simulink model "lab1s2022a"  (R2022b)
settings: Solver=VariableStepAuto  StartTime=0.0  StopTime=Tmdl*0.2  MaxStep=0.001  RelTol=1e-3
undefined symbols (not defined in the file): b12, dfi, J1, J2, k12, Ke, KT, Ra, T1, T2, Ta, Tref, Ua
libraries: slctrlblks x3
settings Model: Creator=81502  LastModifiedBy=86156
settings ModelReferenceCC: EnableRefExpFcnMdlSchedulingChecks=on

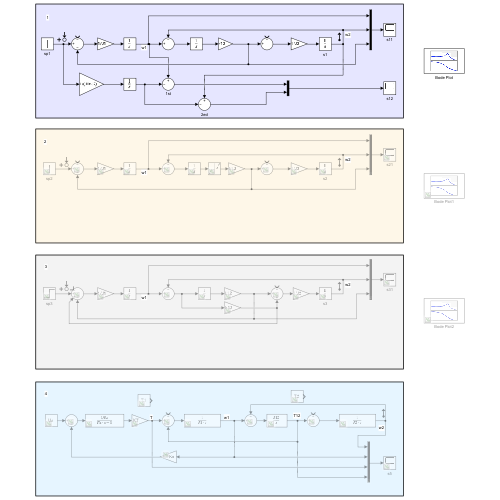
[thumbnail: Simulink's stored preview of the top-level diagram]
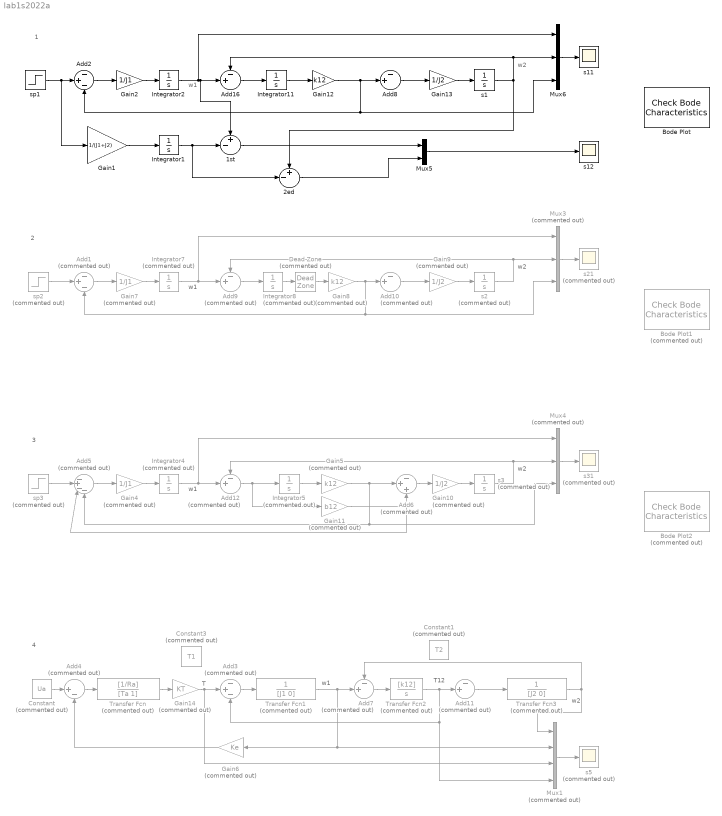
== system lab1s2022a ==
  note: T12
  note: w1
  note: T
  note: 3
  note: 2
  note: 1
  note: w2
  note: w1
  note: w1
  note: w2
  note: w1
  note: w2
  note: 4
  note: w2
  1st : Sum  Inputs=+-|
  2ed : Sum  Inputs=+-|
  Add1 : Sum  Commented=on  Inputs=-+-
  Add{7,9..12} (5 alike) : Sum  Commented=on  Inputs=-+|
  Add16 : Sum  Inputs=-+|
  Add2 : Sum  Inputs=-+-
  Add3 : Sum  Commented=on  Inputs=-+-
  Add4 : Sum  Commented=on  Inputs=|+-
  Add5 : Sum  Commented=on  Inputs=|-+--
  Add6 : Sum  Commented=on  Inputs=-++
  Add8 : Sum  Inputs=-+|
  Bode Plot : slctrlblks/Model Verification/Check Bode  Characteristics  InstantiateOnLoad=on  SaveOperatingPoints=off  LinearizationIOs={'/sp1', 1, 'in', 'off', '';'/s1', 1, 'out', 'off', ''}  LinearizeAt=SnapshotTimes  SnapshotTimes=[0]  TriggerType=rising  SampleTime=auto  RateConversionMethod=zoh  PreWarpFreq=10  UseExactDelayModel=off  UseFullBlockNameLabels=off  UseBusSignalLabels=off  enabled=on  stopWhenAssertionFail=off  export=off  ViewDlgPos=[1264.33333333333 431.666666666667 864 493.333333333333]  OpenViewOnLoad=off  LaunchViewOnOpen=on  FrequencyUnits=rad/s  MagnitudeUnits=dB  PhaseUnits=deg  TimeUnits=seconds  EnableUpperBound=off  UpperBoundFrequencies=[]  UpperBoundMagnitudes=[]  EnableLowerBound=off  LowerBoundFrequencies=[]  LowerBoundMagnitudes=[]
  Bode Plot1 : slctrlblks/Model Verification/Check Bode  Characteristics  Commented=on  InstantiateOnLoad=on  SaveOperatingPoints=off  LinearizationIOs={'/sp2', 1, 'in', 'off', '';'/s2', 1, 'out', 'off', ''}  LinearizeAt=SnapshotTimes  SnapshotTimes=[0]  TriggerType=rising  SampleTime=auto  RateConversionMethod=zoh  PreWarpFreq=10  UseExactDelayModel=off  UseFullBlockNameLabels=off  UseBusSignalLabels=off  enabled=on  stopWhenAssertionFail=off  export=off  ViewDlgPos=[1489 63.6666666666667 620 384]  OpenViewOnLoad=off  LaunchViewOnOpen=on  FrequencyUnits=rad/s  MagnitudeUnits=dB  PhaseUnits=deg  TimeUnits=seconds  EnableUpperBound=off  UpperBoundFrequencies=[]  UpperBoundMagnitudes=[]  EnableLowerBound=off  LowerBoundFrequencies=[]  LowerBoundMagnitudes=[]
  Bode Plot2 : slctrlblks/Model Verification/Check Bode  Characteristics  Commented=on  InstantiateOnLoad=on  SaveOperatingPoints=off  LinearizationIOs={'/sp3', 1, 'in', 'off', '';'/s3', 1, 'out', 'off', ''}  LinearizeAt=SnapshotTimes  SnapshotTimes=[0]  TriggerType=rising  SampleTime=auto  RateConversionMethod=zoh  PreWarpFreq=10  UseExactDelayModel=off  UseFullBlockNameLabels=off  UseBusSignalLabels=off  enabled=on  stopWhenAssertionFail=off  export=off  ViewDlgPos=[1489 63.6666666666667 620 384]  OpenViewOnLoad=off  LaunchViewOnOpen=on  FrequencyUnits=rad/s  MagnitudeUnits=dB  PhaseUnits=deg  TimeUnits=seconds  EnableUpperBound=off  UpperBoundFrequencies=[]  UpperBoundMagnitudes=[]  EnableLowerBound=off  LowerBoundFrequencies=[]  LowerBoundMagnitudes=[]
  Constant : Constant  Commented=on  Value=Ua
  Constant1 : Constant  Commented=on  Value=T2
  Constant3 : Constant  Commented=on  Value=T1
  Dead Zone : DeadZone  Commented=on  LowerValue=-dfi/2  UpperValue=dfi/2
  Gain1 : Gain  Gain=1/(J1+J2)
  Gain10 : Gain  Commented=on  Gain=1/J2
  Gain11 : Gain  Commented=on  Gain=b12
  Gain12 : Gain  Gain=k12
  Gain13 : Gain  Gain=1/J2
  Gain14 : Gain  Commented=on  Gain=KT
  Gain2 : Gain  Gain=1/J1
  Gain4 : Gain  Commented=on  Gain=1/J1
  Gain5 : Gain  Commented=on  Gain=k12
  Gain6 : Gain  Commented=on  Gain=Ke
  Gain7 : Gain  Commented=on  Gain=1/J1
  Gain8 : Gain  Commented=on  Gain=k12
  Gain9 : Gain  Commented=on  Gain=1/J2
  Integrator1 : Integrator
  Integrator11 : Integrator
  Integrator2 : Integrator
  Integrator{4..5,7..8} (4 alike) : Integrator  Commented=on
  Mux1 : Mux  Commented=on
  Mux3 : Mux  Commented=on  Inputs=3
  Mux4 : Mux  Commented=on  Inputs=3
  Mux5 : Mux  Inputs=2
  Mux6 : Mux  Inputs=3
  Transfer Fcn : TransferFcn  Commented=on  Numerator=[1/Ra]  Denominator=[Ta 1]
  Transfer Fcn1 : TransferFcn  Commented=on  Denominator=[J1 0]
  Transfer Fcn2 : TransferFcn  Commented=on  Numerator=[k12]  Denominator=[1 0]
  Transfer Fcn3 : TransferFcn  Commented=on  Denominator=[J2 0]
  s1 : Integrator
  s11 : Scope
  s12 : Scope
  s2 : Integrator  Commented=on
  s21 : Scope  Commented=on
  s3 : Integrator  Commented=on
  s31 : Scope  Commented=on
  s5 : Scope  Commented=on
  sp1 : Step  Time=0.1  After=Tref  SampleTime=0
  sp2 : Step  Commented=on  Time=0.1  After=0.1*Tref  SampleTime=0
  sp3 : Step  Commented=on  Time=0.1  After=Tref  SampleTime=0
  wires:
  s2/1 -> Add9/1, Mux3/2
  Add9/1 -> Integrator8/1
  Gain7/1 -> Integrator7/1
  Add10/1 -> Gain9/1
  Gain8/1 -> Add10/2, Add1/3, Mux3/3
  Gain9/1 -> s2/1
  Add1/1 -> Gain7/1
  Mux3/1 -> s21/1
  Integrator7/1 -> Add9/2, Mux3/1
  sp2/1 -> Add1/2
  Gain5/1 -> Add5/4, Mux4/3, Add6/2
  Mux4/1 -> s31/1
  Gain10/1 -> s3/1
  Gain4/1 -> Integrator4/1
  Add12/1 -> Gain11/1, Integrator5/1
  sp3/1 -> Add5/2
  Integrator5/1 -> Gain5/1
  s3/1 -> Add12/1, Mux4/2
  Add6/1 -> Gain10/1
  Add5/1 -> Gain4/1
  Integrator4/1 -> Add12/2, Mux4/1
  Gain11/1 -> Add6/3, Add5/3
  Add16/1 -> Integrator11/1
  Integrator11/1 -> Gain12/1
  Mux6/1 -> s11/1
  Gain13/1 -> s1/1
  Gain2/1 -> Integrator2/1
  sp1/1 -> Add2/2, Gain1/1
  s1/1 -> 2ed/1, Add16/1, Mux6/2
  Gain12/1 -> Add8/2, Add2/3, Mux6/3
  Add8/1 -> Gain13/1
  1st/1 -> Mux5/1
  2ed/1 -> Mux5/2
  Add2/1 -> Gain2/1
  Gain1/1 -> Integrator1/1
  Integrator1/1 -> 2ed/2, 1st/2
  Integrator2/1 -> Add16/2, 1st/1, Mux6/1
  Mux5/1 -> s12/1
  Dead Zone/1 -> Gain8/1
  Integrator8/1 -> Dead Zone/1
  Add3/1 -> Transfer Fcn1/1
  Add7/1 -> Transfer Fcn2/1
  Gain14/1 -> Add3/2, Mux1/3
  Transfer Fcn2/1 -> Add11/2, Add3/3, Mux1/4
  Constant/1 -> Add4/1
  Mux1/1 -> s5/1
  Transfer Fcn1/1 -> Add7/2, Gain6/1, Mux1/2
  Add4/1 -> Transfer Fcn/1
  Gain6/1 -> Add4/2
  Transfer Fcn/1 -> Gain14/1
  Add11/1 -> Transfer Fcn3/1
  Transfer Fcn3/1 -> Add7/1, Mux1/1
